simulink model "simulink_system"  (R2020a)
settings: Solver=VariableStepAuto  StartTime=0.0  StopTime=5  RelTol=1e-3
values from neighbouring files (symbols this model uses):
  y0 = y1(end,:)    [main.m]    (also in prerun.m = [q10 q20 q30 0   0   0   0]')
settings Model: Creator=none  LastModifiedBy=none

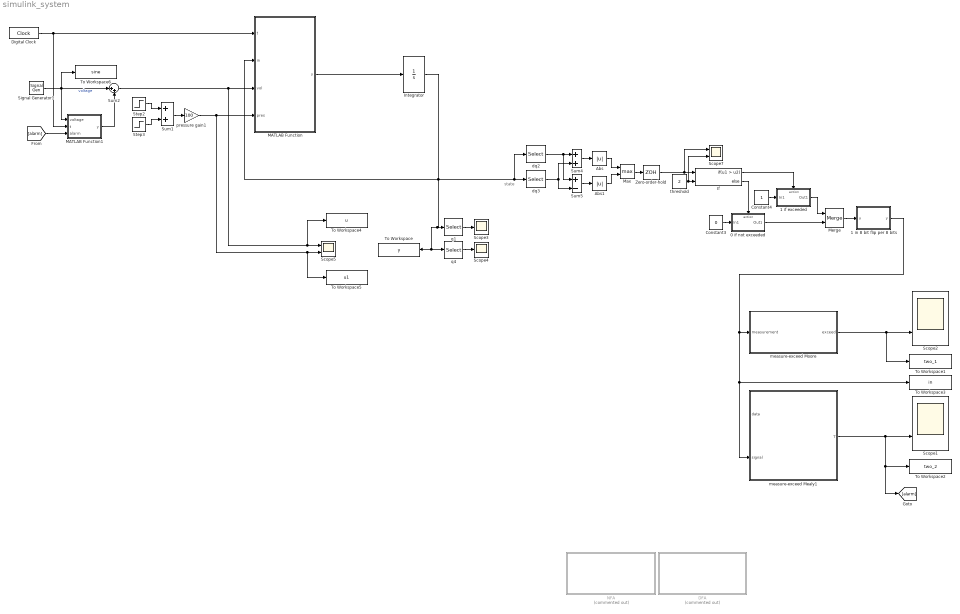
== system simulink_system ==
  note: state
  0 if not exceeded : Subsystem  TreatAsAtomicUnit=on
  1 if exceeded : Subsystem  TreatAsAtomicUnit=on
  1 in 8 bit flip per 8 bits : MATLAB Function  TreatAsAtomicUnit=on
  Abs : Abs
  Abs1 : Abs
  Constant3 : Constant  Value=0
  Constant4 : Constant
  DFA : Stateflow chart  Commented=on  TreatAsAtomicUnit=on
  Digital Clock : DigitalClock  SampleTime=1/10000
  If : If  NumInputs=2  IfExpression=u1 > u2
  Integrator : Integrator  InitialCondition=y0
  MATLAB Function : MATLAB Function  TreatAsAtomicUnit=on
  MATLAB Function1 : MATLAB Function  TreatAsAtomicUnit=on
  Max : MinMax  Function=max  Inputs=2
  Merge : Merge
  NFA : Stateflow chart  Commented=on  TreatAsAtomicUnit=on
  Scope{1..2,5,7} (4 alike) : Scope  NumInputPorts=2
  Scope3 : Scope
  Scope4 : Scope
  Signal Generator1 : SignalGenerator  Amplitude=100
  Step2 : Step  Time=2  SampleTime=0
  Step3 : Step  Time=4  After=-1  SampleTime=0
  Sum1 : Sum
  Sum2 : Sum  Inputs=|++
  Sum4 : Sum
  Sum5 : Sum  Inputs=+-
  To Workspace : ToWorkspace  VariableName=y  SaveFormat=Timeseries  SampleTime=-1
  To Workspace1 : ToWorkspace  VariableName=two_1  SaveFormat=Timeseries  SampleTime=-1
  To Workspace2 : ToWorkspace  VariableName=two_2  SaveFormat=Timeseries  SampleTime=-1
  To Workspace3 : ToWorkspace  VariableName=in  SaveFormat=Timeseries  SampleTime=-1
  To Workspace4 : ToWorkspace  VariableName=u  SaveFormat=Timeseries  SampleTime=-1
  To Workspace5 : ToWorkspace  VariableName=u1  SaveFormat=Timeseries  SampleTime=-1
  To Workspace6 : ToWorkspace  VariableName=sine  SaveFormat=Timeseries  SampleTime=-1
  Zero-order-hold : ZeroOrderHold  SampleTime=1/100
  dq2 : Selector  InputPortWidth=7  IndexOptions=Index vector (dialog)  Indices=5  OutputSizes=1
  dq3 : Selector  InputPortWidth=7  IndexOptions=Index vector (dialog)  Indices=6  OutputSizes=1
  measure-exceed Mealy1 : Stateflow chart  TreatAsAtomicUnit=on
  measure-exceed Moore : Stateflow chart  TreatAsAtomicUnit=on
  pressure gain1 : Gain  Gain=100
  q1 : Selector  InputPortWidth=7  IndexOptions=Index vector (dialog)  Indices=[1 2 3]  OutputSizes=1
  q4 : Selector  InputPortWidth=7  IndexOptions=Index vector (dialog)  Indices=[4 5 6]  OutputSizes=1
  threshold : Constant  Value=2
  wires:
  measure-exceed Moore/1(exceed) -> Scope2/2, To Workspace1/1
  Digital Clock/1 -> MATLAB Function1/2(t), MATLAB Function/1(t)
  MATLAB Function/1(y) -> Integrator/1
  Step2/1 -> Sum1/1
  Step3/1 -> Sum1/2
  Sum1/1 -> pressure gain1/1
  pressure gain1/1 -> To Workspace5/1, Scope5/2, MATLAB Function/4(pres)
  measure-exceed Mealy1/1(T) -> [alarm], To Workspace2/1, Scope1/2
  dq2/1 -> Sum5/1, Sum4/1
  dq3/1 -> Sum5/2, Sum4/2
  Max/1 -> Zero-order-hold/1
  threshold/1 -> Scope7/2, If/2
  Zero-order-hold/1 -> Scope7/1, If/1
  Sum4/1 -> Abs/1
  Sum5/1 -> Abs1/1
  Abs1/1 -> Max/2
  Abs/1 -> Max/1
  If/1 -> 1 if exceeded/Action
  Constant4/1 -> 1 if exceeded/1(In1)
  If/2 -> 0 if not exceeded/Action
  Constant3/1 -> 0 if not exceeded/1(In1)
  0 if not exceeded/1(Out1) -> Merge/2
  1 if exceeded/1(Out1) -> Merge/1
  ? -> ?
  q4/1 -> Scope4/1
  q1/1 -> Scope3/1
  Integrator/1 -> dq3/1, dq2/1, MATLAB Function/2(in), To Workspace/1, q4/1, q1/1
  Merge/1 -> 1 in 8 bit flip per 8 bits/1(u)
  [alarm] -> MATLAB Function1/3(alarm)
  Sum2/1 -> To Workspace4/1, Scope5/1, MATLAB Function/3(vol)
  Signal Generator1/1 -> To Workspace6/1, MATLAB Function1/1(voltage), Sum2/1  "voltage"
  MATLAB Function1/1(y) -> Sum2/2
  1 in 8 bit flip per 8 bits/1(y) -> To Workspace3/1, measure-exceed Mealy1/2(signal), measure-exceed Moore/1(measurement)

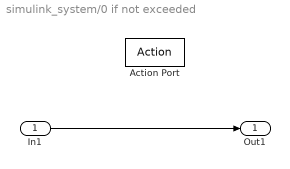
== system simulink_system/0 if not exceeded ==
  In1 : Inport
  Action Port : ActionPort  ActionPortLabel=else
  Out1 : Outport
  wires:
  In1/1 -> Out1/1

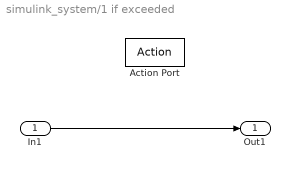
== system simulink_system/1 if exceeded ==
  In1 : Inport
  Action Port : ActionPort  ActionPortLabel=if(u1 > u2)
  Out1 : Outport
  wires:
  In1/1 -> Out1/1

== stateflow chart simulink_system/DFA ==
  settings: stateMachineType=MOORE_MACHINE
  state ? [group]
    state a103
      1111
      1000
      _
      1111    1111
      0000    0001
      _
      1111
      0010
      _
      1111
      0100
  state ? [group]
    state a73
      0111
      1000
      _
      0111    0111
      0000    0001
      _
      0111
      0010
      _
      0111
      0100
  state a100
    0111
    0100
    _
    0111
    0000
    _
    0111
    0001
    _
    0111
    0010
  state a71
    0011
    0100
    _
    0011
    0000
    _
    0011
    0001
    _
    0011
    0010
  state ? [group]
    state a74
      0110
      1000
      _
      0110    0110
      0000    0001
      _
      0110
      0010
      _
      0110
      0100
  state ? [group]
    state a105
      1110
      1000
      _
      1110    1110
      0000    0001
      _
      1110
      0010
      _
      1110
      0100
  state a69
    0001
    0010
    _
    0001
    0000
    _
    0001
    0001
  state a107
    0011
    0010
    _
    0011
    0000
    _
    0011
    0001
  state ? [group]
    state a97
      1101
      1000
      _
      1101    1101
      0000    0001
      _
      1101
      0010
      _
      1101
      0100
  state ? [group]
    state a85
      0101
      1000
      _
      0101    0101
      0000    0001
      _
      0101
      0010
      _
      0101
      0100
  state a101
    0110
    0100
    _
    0110
    0000
    _
    0110
    0001
    _
    0110
    0010
  state a72
    0010
    0100
    _
    0010
    0000
    _
    0010
    0001
    _
    0010
    0010
  state ? [group]
    state a108
      1100
      1000
      _
      1100    1100
      0000    0001
      _
      1100
      0010
      _
      1100
      0100
  state a86
    0100
    1000
    _
    0100    0100
    0000    0001
    _
    0100
    0010
    _
    0100
    0100
  state a70
    0001
    0001
    _
    0001
    0000
  state a52
    0000
    0001
    _
    0000
    0000
  state a47
    0000
    0000
  state ? [group]
    state a90
      0011
      1000
      _
      0011    0011
      0000    0001
      _
      0011
      0010
      _
      0011
      0100
  state ? [group]
    state a98
      1011
      1000
      _
      1011    1011
      0000    0001
      _
      1011
      0010
      _
      1011
      0100
  state a99
    0101
    0100
    _
    0101
    0000
    _
    0101
    0001
    _
    0101
    0010
  state a88
    0001
    0100
    _
    0001
    0000
    _
    0001
    0001
    _
    0001
    0010
  state ? [group]
    state a106
      1010
      1000
      _
      1010    1010
      0000    0001
      _
      1010
      0010
      _
      1010
      0100
  state a91
    0010
    1000
    _
    0010    0010
    0000    0001
    _
    0010
    0010
    _
    0010
    0100
  state a92
    0000
    0010
    _
    0000
    0000
    _
    0000
    0001
  state a102
    0010
    0010
    _
    0010
    0000
    _
    0010
    0001
  state ? [group]
    state a104
      1001
      1000
      _
      1001    1001
      0000    0001
      _
      1001
      0010
      _
      1001
      0100
  state a93
    0001
    1000
    _
    0001    0001
    0000    0001
    _
    0001
    0010
    _
    0001
    0100
  state a95
    0100
    0100
    _
    0100
    0000
    _
    0100
    0001
    _
    0100
    0010
  state a89
    0000
    0100
    _
    0000
    0000
    _
    0000
    0001
    _
    0000
    0010
  state a96
    1000
    1000
    _
    1000    1000
    0000    0001
    _
    1000
    0010
    _
    1000
    0100
  state a94
    0000
    1000
    _
    0000    0000
    0000    0001
    _
    0000
    0010
    _
    0000
    0100
  a100 -> a103 [order 1] : [1]
  a71 -> a73 [order 1] : [1]
  a100 -> a105 [order 2] : [0]
  a107 -> a100 [order 1] : [1]
  a69 -> a71 [order 1] : [1]
  a71 -> a74 [order 2] : [0]
  a52 -> a69 [order 1] : [1]
  a70 -> a107 [order 2] : [1]
  a69 -> a72 [order 2] : [0]
  a101 -> a97 [order 1] : [1]
  a107 -> a101 [order 2] : [0]
  a72 -> a85 [order 1] : [1]
  a72 -> a86 [order 2] : [0]
  a101 -> a108 [order 2] : [0]
  a47 -> a52 [order 1] : [0]
  a47 -> a70 [order 2] : [1]
  a52 -> a92 [order 2] : [0]
  a70 -> a102 [order 1] : [0]
  a99 -> a98 [order 1] : [1]
  a88 -> a90 [order 1] : [1]
  a102 -> a99 [order 1] : [1]
  a92 -> a88 [order 1] : [1]
  a99 -> a106 [order 2] : [0]
  a88 -> a91 [order 2] : [0]
  a92 -> a89 [order 2] : [0]
  a102 -> a95 [order 2] : [0]
  a95 -> a104 [order 1] : [1]
  a89 -> a93 [order 1] : [1]
  a89 -> a94 [order 2] : [0]
  a95 -> a96 [order 2] : [0]

== stateflow chart simulink_system/measure-exceed Moore ==
  settings: stateMachineType=MOORE_MACHINE
  state Name
    exceed=0
  state Name1
    exceed=0
  state Name8
    exceed=1
  state Name2
    exceed=0
  state Name3
    exceed=0
  state Name4
    exceed=0
  state Name5
    exceed=0
  state Name6
    exceed=0
  state Name7
    exceed=0
  (default) -> Name
  Name -> Name [order 2] : [measurement==0]
  Name1 -> Name8 [order 1] : [measurement==1]
  Name -> Name1 [order 1] : [measurement==1]
  Name1 -> Name2 [order 2] : [measurement==0]
  Name5 -> Name8 [order 1] : [measurement==1]
  Name7 -> Name8 : [measurement==1]
  Name2 -> Name8 [order 2] : [measurement==1]
  Name6 -> Name8 [order 1] : [measurement==1]
  Name4 -> Name8 [order 2] : [measurement==1]
  Name3 -> Name8 [order 2] : [measurement==1]
  Name2 -> Name3 [order 1] : [measurement==0]
  Name3 -> Name4 [order 1] : [measurement==0]
  Name4 -> Name5 [order 1] : [measurement==0]
  Name5 -> Name6 [order 2] : [measurement==0]
  Name6 -> Name7 [order 2] : [measurement==0]
  data: measurement input; exceed output

== stateflow chart simulink_system/measure-exceed Mealy1 ==
  settings: stateMachineType=MEALY_MACHINE  initializeOutput=1
  state checking for unsure [group]
    state a5
    state a4
    state a6
    state a
    state a13
    state a14
    state a12
    state a1
    state a3
    a5 -> a5 [order 2] : [signal==1&&one~=5&&cnt!=7]{cnt=cnt+1,one=one+1,T=1}
    a4 -> a5 [order 2] : [signal==1&&cnt!=7]{cnt=cnt+1,one=one+1,T=1}
    a14 -> a5 [order 1] : [signal==1&&cnt!=7]{cnt=cnt+1,one=one+1,T=1}
    a -> a4 [order 2] : [signal==1&&cnt!=7]{cnt=cnt+1,one=one+1,T=0}
    a4 -> a6 [order 1] : [signal==0&&cnt!=7]{cnt=cnt+1,T=1}
    a6 -> a6 [order 2] : [signal==1&&one!=5&&cnt!=7]{cnt=cnt+1,one=one+1,T=1}
    a14 -> a6 [order 3] : [signal==0&&cnt!=7]{cnt=cnt+1,T=1}
    a -> a1 [order 1] : [signal==0&&cnt!=7]{cnt=cnt+1,T=0}
    a12 -> a13 [order 1] : [signal==1&&cnt!=7]{cnt=cnt+1,one=one+1,T=0}
    a13 -> a14 [order 1] : [signal==1&&cnt!=7]{cnt=cnt+1,one=one+1,T=1}
    a13 -> a1 [order 3] : [signal==0&&cnt!=7]{cnt=cnt+1,one=one+1,T=0}
    a3 -> a3 [order 1] : [signal==1&&cnt!=7]{cnt=cnt+1,one=one+1,T=1}
    a1 -> a3 [order 2] : [signal==1&&cnt!=7]{cnt=cnt+1,one=one+1,T=1}
    a1 -> a12 [order 1] : [signal==0&&cnt!=7]{cnt=cnt+1,T=0}
    a12 -> a12 [order 2] : [signal==0&&cnt!=7]{cnt=cnt+1,T=0}
  state sure [group]
    state a19
    state a20
    state a21
    a19 -> a19 [order 1] : [signal==1&&cnt!=7]{cnt=cnt+1,one=one+1,T=2}
    a19 -> a19 [order 2] : [signal==0&&cnt!=7]{cnt=cnt+1,T=2}
    a20 -> a20 [order 1] : [signal==1&&cnt!=7]{cnt=cnt+1,one=one+1,T=2}
    a20 -> a20 [order 2] : [signal==0&&cnt!=7]{cnt=cnt+1,T=2}
    a21 -> a21 [order 1] : [signal==1&&cnt!=7]{cnt=cnt+1,one=one+1,T=2}
    a21 -> a21 [order 2] : [signal==0&&cnt!=7]{cnt=cnt+1,T=2}
  state unsure and not going to be sure [group]
    state a16
    state a17
    state a18
    a16 -> a16 [order 1] : [signal==1&&cnt!=7]{cnt=cnt+1,one=one+1,T=1}
    a16 -> a16 [order 2] : [signal==0&&cnt!=7]{cnt=cnt+1,T=1}
    a17 -> a17 [order 1] : [signal==1&&cnt!=7]{cnt=cnt+1,one=one+1,T=1}
    a17 -> a17 [order 2] : [signal==0&&cnt!=7]{cnt=cnt+1,T=1}
    a18 -> a18 [order 1] : [signal==1&&cnt!=7]{cnt=cnt+1,one=one+1,T=1}
    a18 -> a18 [order 2] : [signal==0&&cnt!=7]{cnt=cnt+1,T=1}
  state Begin
  a21 -> Begin [order 3] : [(signal==1||signal==0)&&cnt==7]{cnt=0,one=0,T=2}
  a20 -> Begin [order 3] : [(signal==1||signal==0)&&cnt==7]{cnt=0,one=0,T=2}
  a19 -> Begin [order 3] : [(signal==1||signal==0)&&cnt==7]{cnt=0,one=0,T=2}
  a6 -> Begin [order 4] : [(signal==1||signal==0)&&cnt==7]{cnt=0,one=0,T=1}
  a5 -> Begin [order 4] : [(signal==1||signal==0)&&cnt==7]{cnt=0,one=0,T=1}
  a5 -> a19 [order 3] : [signal==1&&one==5&&cnt~=7]{cnt=cnt+1,one=one+1,T=2}
  a5 -> a16 [order 1] : [signal==0&&cnt!=7]{cnt=cnt+1,T=1}
  a4 -> Begin [order 3] : [(signal==1||signal==0)&&cnt==7]{cnt=0,one=0,T=0}
  a16 -> Begin [order 3] : [(signal==1||signal==0)&&cnt==7]{cnt=0,one=0,T=1}
  a14 -> Begin [order 2] : [(signal==1||signal==0)&&cnt==7]{cnt=0,one=0,T=0}
  a13 -> Begin [order 2] : [(signal==1||signal==0)&&cnt==7]{cnt=0,one=0,T=0}
  a6 -> a20 [order 3] : [signal==1&&one==5&&cnt!=7]{cnt=cnt+1,one=one+1,T=2}
  a6 -> a17 [order 1] : [signal==0&&cnt!=7]{cnt=cnt+1,T=1}
  Begin -> a [order 1] : [signal==1]{cnt=1,one=one+1,T=0}
  (default) -> Begin : {cnt=0,one=0,T=0}
  Begin -> a12 [order 2] : [signal==0]{cnt=1,T=0}
  a1 -> Begin [order 3] : [(signal==1||signal==0)&&cnt==7]{cnt=0,one=0,T=0}
  a12 -> Begin [order 3] : [(signal==1||signal==0)&&cnt==7]{cnt=0,one=0,T=0}
  a17 -> Begin [order 3] : [(signal==1||signal==0)&&cnt==7]{cnt=0,one=0,T=1}
  a18 -> Begin [order 3] : [(signal==1||signal==0)&&cnt==7]{cnt=0,one=0,T=1}
  a3 -> Begin [order 4] : [(signal==1||signal==0)&&cnt==7]{cnt=0,one=0,T=1}
  a3 -> a21 [order 2] : [signal==1&&one==5&&cnt!=7]{cnt=cnt+1,one=one+1,T=2}
  a3 -> a18 [order 3] : [signal==0&&cnt!=7]{cnt=cnt+1,T=1}
  data: data input; signal input; T output double; cnt local double; one local double

== matlab function simulink_system/MATLAB Function ==
  data: t input; y output; in input; vol input; pres input
function y = fcn(t,in,vol,pres)
y = evaluateEoM(t,in,vol,pres);

== matlab function simulink_system/MATLAB Function1 ==
  settings: updateMethod=DISCRETE
  data: voltage input; t input; alarm input; y output
function y = fcn(voltage, t, alarm)
persistent tUntil
if isempty(tUntil)
    tUntil = 0;
end

if alarm == 2
    tUntil = t + 2;
end
    

if t <= tUntil
    y = -voltage;
else 
    y = 0;
end

== matlab function simulink_system/1 in 8 bit flip per 8 bits ==
  data: u input; y output
function y = fcn(u)
persistent count randomized
if isempty(count)
    count = 1;
    randomized = 0;
elseif count == 8
    count = 1;
    randomized = 0;
else
    count = count + 1;
end

if randomized == 0
    flip = rand(1) < 1/8;
    if flip && u == 1
        u = 0;
    elseif flip && u == 0
        u = 1;
    end
    randomized = 1;
end
y = u;

== stateflow chart simulink_system/NFA ==
  settings: stateMachineType=MOORE_MACHINE
  state ? [group]
    state a43
      1111
      0100
    state a41
      0111
      0010
    state a44
      1110
      0100
    state a5
      0011
      0001
    state a47
      1101
      0100
    state a42
      0110
      0010
    state a46
      1100
      0100
    state a51
      1011
      0100
    state a49
      0101
      0010
    state a53
      1010
      0100
    state a8
      0010
      0001
    state a48
      1001
      0100
    state a50
      0100
      0010
    state a52
      1000
      0100
    state ? [group]
      state a70
        1111
        0010
      state a66
        0111
        0001
      state a71
        1110
        0010
      state a73
        1101
        0010
      state a67
        0110
        0001
      state a7
        0011
        0000
      state a72
        1100
        0010
      state ? [group]
        state a74
          1111
          0001
        state a75
          1110
          0001
        state a68
          0111
          0000
        state a76
          1111
          0000
        state a77
          1110
          0000
        state a81
          0111
          0001
        state a78
          0110
          0001
        state a69
          0110
          0000
        state a80
          0111
          0000
        state a79
          0110
          0000
        a68 -> a74 [order 1] : [1,1]
        a68 -> a75 [order 2] : [0,1]
        a68 -> a76 [order 3] : [1,0]
        a68 -> a77 [order 4] : [0,0]
        a69 -> a81 [order 1] : [1,1]
        a69 -> a78 [order 4] : [0,1]
        a69 -> a80 [order 3] : [1,0]
        a69 -> a79 [order 2] : [0,0]
      state a96
        1011
        0010
      state a97
        0101
        0001
      state a82
        1010
        0010
      state a92
        1001
        0010
      state a83
        0100
        0001
      state a6
        0010
        0000
      state a91
        1000
        0010
      state ? [group]
        state a95
          1011
          0001
        state a86
          1010
          0001
        state a94
          0101
          0000
        state a93
          1011
          0000
        state a87
          1010
          0000
        state a85
          1001
          0001
        state a88
          1000
          0001
        state a84
          0100
          0000
        state a89
          1001
          0000
        state a90
          1000
          0000
        a94 -> a95 [order 1] : [1,1]
        a94 -> a86 [order 2] : [0,1]
        a94 -> a93 [order 3] : [1,0]
        a94 -> a87 [order 4] : [0,0]
        a84 -> a85 [order 1] : [1,1]
        a84 -> a88 [order 4] : [0,1]
        a84 -> a89 [order 3] : [1,0]
        a84 -> a90 [order 2] : [0,0]
      a66 -> a70 [order 1] : [1,0]
      a7 -> a66 [order 1] : [1,1]
      a66 -> a71 [order 2] : [0,0]
      a67 -> a73 [order 1] : [1,0]
      a7 -> a67 [order 2] : [0,1]
      a67 -> a72 [order 2] : [0,0]
      a7 -> a68 [order 3] : [1,0]
      a7 -> a69 [order 4] : [0,0]
      a97 -> a96 [order 1] : [1,0]
      a6 -> a97 [order 1] : [1,1]
      a97 -> a82 [order 2] : [0,0]
      a83 -> a92 [order 1] : [1,0]
      a6 -> a83 [order 3] : [0,1]
      a83 -> a91 [order 2] : [0,0]
      a6 -> a94 [order 2] : [1,0]
      a6 -> a84 [order 4] : [0,0]
    state a2
      0001
      0000
    state a61
      0111
      0100
    state a59
      0011
      0010
    state a63
      0110
      0100
    state a40
      0001
      0001
    state a58
      0101
      0100
    state a60
      0010
      0010
    state a62
      0100
      0100
    state a65
      0011
      0100
    state a57
      0001
      0010
    state a64
      0010
      0100
    state a39
      0000
      0001
    state a54
      0001
      0100
    state a55
      0000
      0010
    state a56
      0000
      0100
    state ? [group]
      state a128
        0111
        0010
      state a129
        0011
        0001
      state a98
        0110
        0010
      state a120
        0101
        0010
      state a99
        0010
        0001
      state a124
        0001
        0000
      state a119
        0100
        0010
      state ? [group]
        state a125
          0111
          0001
        state a105
          0110
          0001
        state a122
          0011
          0000
        state a121
          0111
          0000
        state a106
          0110
          0000
        state a102
          0101
          0001
        state a110
          0100
          0001
        state a101
          0010
          0000
        state a112
          0101
          0000
        state a118
          0100
          0000
        a122 -> a125 [order 1] : [1,1]
        a122 -> a105 [order 2] : [0,1]
        a122 -> a121 [order 3] : [1,0]
        a122 -> a106 [order 4] : [0,0]
        a101 -> a102 [order 1] : [1,1]
        a101 -> a110 [order 4] : [0,1]
        a101 -> a112 [order 3] : [1,0]
        a101 -> a118 [order 2] : [0,0]
      state a103
        0011
        0010
      state a104
        0001
        0001
      state a113
        0010
        0010
      state a127
        0001
        0010
      state a130
        0000
        0001
      state a123
        0000
        0000
      state a108
        0000
        0010
      state ? [group]
        state a126
          0011
          0001
        state a117
          0010
          0001
        state a115
          0001
          0000
        state a114
          0011
          0000
        state a100
          0010
          0000
        state a131
          0001
          0001
        state a116
          0000
          0001
        state a111
          0000
          0000
        state a109
          0001
          0000
        state a107
          0000
          0000
        a115 -> a126 [order 1] : [1,1]
        a115 -> a117 [order 2] : [0,1]
        a115 -> a114 [order 3] : [1,0]
        a115 -> a100 [order 4] : [0,0]
        a111 -> a131 [order 1] : [1,1]
        a111 -> a116 [order 4] : [0,1]
        a111 -> a109 [order 3] : [1,0]
        a111 -> a107 [order 2] : [0,0]
      a129 -> a128 [order 1] : [1,0]
      a124 -> a129 [order 1] : [1,1]
      a129 -> a98 [order 2] : [0,0]
      a99 -> a120 [order 1] : [1,0]
      a124 -> a99 [order 2] : [0,1]
      a99 -> a119 [order 2] : [0,0]
      a124 -> a122 [order 3] : [1,0]
      a124 -> a101 [order 4] : [0,0]
      a104 -> a103 [order 1] : [1,0]
      a123 -> a104 [order 1] : [1,1]
      a104 -> a113 [order 2] : [0,0]
      a130 -> a127 [order 1] : [1,0]
      a123 -> a130 [order 3] : [0,1]
      a130 -> a108 [order 2] : [0,0]
      a123 -> a115 [order 2] : [1,0]
      a123 -> a111 [order 4] : [0,0]
    state a4
      0000
      0000
    a41 -> a43 [order 1] : [1,0]
    a5 -> a41 [order 1] : [1,0]
    a41 -> a44 [order 2] : [0,0]
    a2 -> a5 [order 1] : [1,1]
    a5 -> a42 [order 2] : [0,0]
    a42 -> a47 [order 2] : [1,0]
    a42 -> a46 [order 1] : [0,0]
    a49 -> a51 [order 1] : [1,0]
    a8 -> a49 [order 1] : [1,0]
    a49 -> a53 [order 2] : [0,0]
    a2 -> a8 [order 4] : [0,1]
    a8 -> a50 [order 2] : [0,0]
    a50 -> a48 [order 2] : [1,0]
    a50 -> a52 [order 1] : [0,0]
    a2 -> a7 [order 3] : [1,0]
    a2 -> a6 [order 2] : [0,0]
    a59 -> a61 [order 1] : [1,0]
    a40 -> a59 [order 1] : [1,0]
    a59 -> a63 [order 2] : [0,0]
    a4 -> a40 [order 1] : [1,1]
    a40 -> a60 [order 2] : [0,0]
    a60 -> a58 [order 2] : [1,0]
    a60 -> a62 [order 1] : [0,0]
    a57 -> a65 [order 1] : [1,0]
    a39 -> a57 [order 1] : [1,0]
    a57 -> a64 [order 2] : [0,0]
    a4 -> a39 [order 2] : [0,1]
    a39 -> a55 [order 2] : [0,0]
    a55 -> a54 [order 2] : [1,0]
    a55 -> a56 [order 1] : [0,0]
    a4 -> a124 [order 4] : [1,0]
    a4 -> a123 [order 3] : [0,0]
  state a17
    1111
    1000
  state a18
    1110
    1000
  state a14
    0111
    0100
  state a11
    0011
    0010
  state a13
    0110
    0100
  state a19
    1101
    1000
  state a20
    1100
    1000
  state a22
    1111
    1000
  state a3
    0001
    0001
  state a21
    1110
    1000
  state a15
    0101
    0100
  state a12
    0010
    0010
  state a24
    1001
    1000
  state a16
    0100
    0100
  state a23
    1000
    1000
  state a34
    0111
    1000
  state a26
    0110
    1000
  state a28
    0011
    0100
  state a9
    0001
    0010
  state a31
    0010
    0100
  state a36
    0101
    1000
  state a35
    0100
    1000
  state a32
    0111
    1000
  state a1
    0000
    0001
  state a33
    0110
    1000
  state a25
    0001
    0100
  state a10
    0000
    0010
  state a27
    0001
    1000
  state a30
    0000
    0100
  state a
    0000
    0000
  state a29
    0000
    1000
  a -> a2 [order 2] : [1,0]
  a14 -> a17 [order 1] : [1,0]
  a11 -> a14 [order 1] : [1,0]
  a14 -> a18 [order 2] : [0,0]
  a3 -> a11 [order 1] : [1,0]
  a13 -> a19 [order 1] : [1,0]
  a11 -> a13 [order 2] : [0,0]
  a13 -> a20 [order 2] : [0,0]
  a15 -> a22 [order 1] : [1,0]
  a -> a3 [order 3] : [1,1]
  a3 -> a12 [order 2] : [0,0]
  a15 -> a21 [order 2] : [0,0]
  a12 -> a15 [order 1] : [1,0]
  a12 -> a16 [order 2] : [0,0]
  a16 -> a24 [order 1] : [1,0]
  a16 -> a23 [order 2] : [0,0]
  a28 -> a34 [order 1] : [1,0]
  a9 -> a28 [order 1] : [1,0]
  a28 -> a26 [order 2] : [0,0]
  a1 -> a9 [order 1] : [1,0]
  a31 -> a36 [order 1] : [1,0]
  a9 -> a31 [order 2] : [0,0]
  a31 -> a35 [order 2] : [0,0]
  a25 -> a32 [order 1] : [1,0]
  a -> a1 [order 1] : [0,1]
  a1 -> a10 [order 2] : [0,0]
  a25 -> a33 [order 2] : [0,0]
  a10 -> a25 [order 1] : [1,0]
  a10 -> a30 [order 2] : [0,0]
  a30 -> a27 [order 1] : [1,0]
  a30 -> a29 [order 2] : [0,0]
  a -> a4 [order 4] : [0,0]
